simulink model "controllo_ottimo_PID"  (R2026a)
settings: Solver=VariableStepAuto  StopTime=30
values from neighbouring files (symbols this model uses):
  A = [0 0 1 0; 0 0 0 1; -2.517 0 -10.915 0; 0 0 0 0]    [sistema_lineare.m]
  B = [0 0; 0 0; 21.83 0; 0 1.236]    [sistema_lineare.m]
  C = [1 0 0 0; 0 1 0 0; 0 0 1 0; 0 0 0 1]    [sistema_lineare.m]
  D = [0 0; 0 0; 0 0; 0 0]    [sistema_lineare.m]
  u_regime = pinv(Bd) * (I - Ad) * x_f    [CONTROLLO_OTTIMO_discretizzazione_feedforward.m]
  u_star = inv(W)*Rd'*inv(Rd*inv(W)*Rd')*(x_f - Ad^n*x_0)    [CONTROLLO_OTTIMO_discretizzazione_feedforward.m]
  x_0 = [0.117; 0; 0; 0]    [CONTROLLO_OTTIMO_discretizzazione_feedforward.m]
undefined symbols (not defined in the file or in its folder): Ad, Bd
libraries: slpidlib x4
settings Model: Creator=user  LastModifiedBy=user

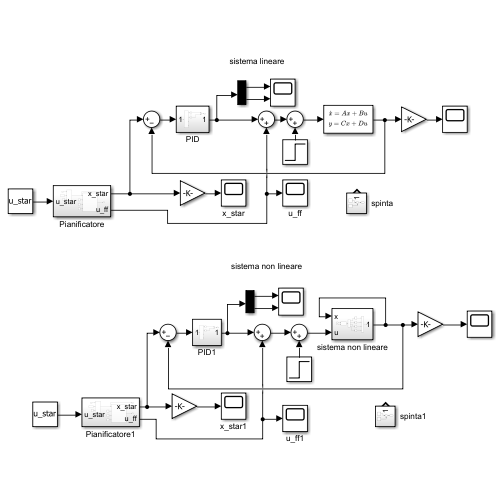
[thumbnail: Simulink's stored preview of the top-level diagram]
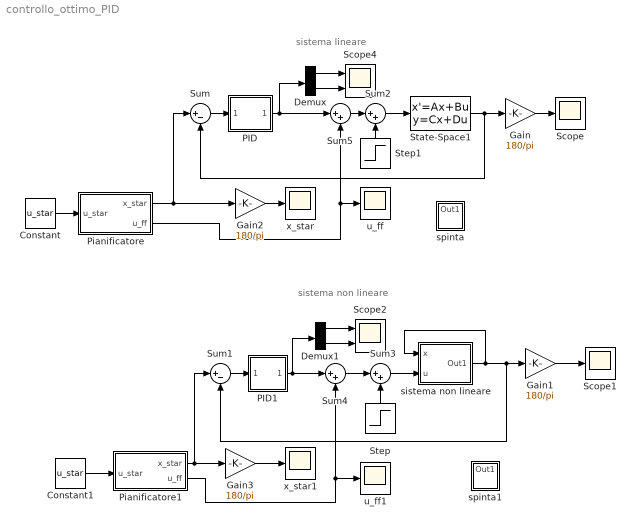
== system controllo_ottimo_PID ==
  note: sistema lineare
  note: sistema non lineare
  Constant : Constant  Value=u_star
  Constant1 : Constant  Value=u_star
  Demux : Demux  Outputs=2
  Demux1 : Demux  Outputs=2
  Gain{,1..3} (4 alike) : Gain  Gain=180/pi
  PID : Subsystem
  PID1 : Subsystem
  Pianificatore : Subsystem
  Pianificatore1 : Subsystem
  Scope : Scope
      settings: Title=angoli e velocità angolari  ActiveDisplayYMinimum=-19.863928702549515  ActiveDisplayYMaximum=100.91969713509383
  Scope1 : Scope
      settings: Title=angoli e velocità angolari  ActiveDisplayYMinimum=-19.863928702549515  ActiveDisplayYMaximum=100.91969713509383  DataLoggingVariableName=ScopeData4
  Scope2 : Scope  NumInputPorts=2
      settings: ActiveDisplayYMinimum=-3.9476866423630206  ActiveDisplayYMaximum=12.694242209293055  DataLoggingVariableName=ScopeData3
  Scope4 : Scope  NumInputPorts=2
      settings: ActiveDisplayYMinimum=-3.9476866423630206  ActiveDisplayYMaximum=12.694242209293055  DataLoggingVariableName=ScopeData6
  State-Space1 : StateSpace  A=A  B=B  C=C  D=D  InitialCondition=[0.117;0;0;0]
  Step : Step  Time=5  FinalValue=0.1  SampleTime=0
  Step1 : Step  Time=5  SampleTime=0
  Sum : Sum  Inputs=|+-
  Sum1 : Sum  Inputs=|+-
  Sum{2..5} (4 alike) : Sum  Inputs=|++
  sistema non lineare : Subsystem
  spinta : Subsystem
  spinta1 : Subsystem
  u_ff : Scope
      settings: Title=u_ff  ActiveDisplayYMinimum=-0.76735028378378445  ActiveDisplayYMaximum=0.87981383783783862
  u_ff1 : Scope
      settings: Title=u_ff  ActiveDisplayYMinimum=-0.70558162922297274  ActiveDisplayYMaximum=1.6384596207770272
  x_star : Scope
      settings: Title=x_star  ActiveDisplayYMinimum=-96.1931  ActiveDisplayYMaximum=305.783  DataLoggingVariableName=ScopeData2
  x_star1 : Scope
      settings: Title=x_star  ActiveDisplayYMinimum=-96.1931  ActiveDisplayYMaximum=305.783  DataLoggingVariableName=ScopeData2
  wires:
  Sum/1 -> PID/1(In1)
  Gain/1 -> Scope/1
  State-Space1/1 -> Sum/2, Gain/1
  Pianificatore1/2(u_ff) -> u_ff1/1, Sum4/2
  Constant1/1 -> Pianificatore1/1(u_star)
  Gain3/1 -> x_star1/1
  sistema non lineare/1(Out1) -> Gain1/1, Sum1/2, sistema non lineare/1(x)
  Sum1/1 -> PID1/1(In1)
  Pianificatore1/1(x_star) -> Gain3/1, Sum1/1
  PID1/1(Out1) -> Sum4/1, Demux1/1
  PID/1(Out1) -> Sum5/1, Demux/1
  Pianificatore/1(x_star) -> Gain2/1, Sum/1
  Gain2/1 -> x_star/1
  Sum4/1 -> Sum3/1
  Sum5/1 -> Sum2/1
  Demux/1 -> Scope4/1
  Demux/2 -> Scope4/2
  Demux1/1 -> Scope2/1
  Demux1/2 -> Scope2/2
  Step1/1 -> Sum2/2
  Step/1 -> Sum3/2
  Pianificatore/2(u_ff) -> Sum5/2, u_ff/1
  Constant/1 -> Pianificatore/1(u_star)
  Sum2/1 -> State-Space1/1
  Sum3/1 -> sistema non lineare/2(u)
  Gain1/1 -> Scope1/1

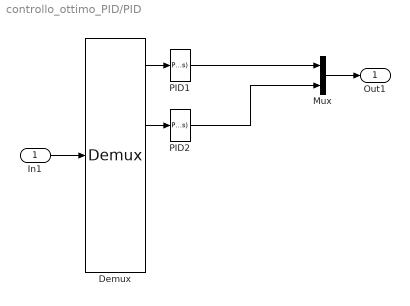
== system controllo_ottimo_PID/PID ==
  In1 : Inport
  Demux : Demux
  Mux : Mux  Inputs=2
  PID1 : slpidlib/PID Controller  Controller=PID  Form=Parallel  TimeDomain=Continuous-time  UseExternalTs=off  SampleTime=-1  IntegratorMethod=Forward Euler  FilterMethod=Forward Euler  ControllerParametersSource=internal  P=2.11205018237787  I=1.49141592854366  UseKiTs=off  D=0.250048510902589  UseExternalDerivativeSource=off  N=10  UseFilter=on  TunerSelectOption=Transfer Function Based (PID Tuner App)  InitialConditionSource=internal  InitialConditionForIntegrator=0  InitialConditionForFilter=0  DifferentiatorICPrevScaledInput=0  ExternalReset=none  TrackingMode=off  Kt=1  LimitOutput=off  SatLimitsSource=internal  UpperSaturationLimit=inf  LowerSaturationLimit=-inf  LinearizeAsGain=on  AntiWindupMode=none  Kb=1  LimitIntegrator=off  UpperIntegratorSaturationLimit=inf  LowerIntegratorSaturationLimit=-inf  POutMin=[]  POutMax=[]  IOutMin=[]  IOutMax=[]  DOutMin=[]  DOutMax=[]  NOutMin=[]  NOutMax=[]  SumOutMin=[]  SumOutMax=[]  SaturationOutMin=[]  SaturationOutMax=[]  PParamMin=[]  PParamMax=[]  IParamMin=[]  IParamMax=[]  DParamMin=[]  DParamMax=[]  NParamMin=[]  NParamMax=[]  KbParamMin=[]  KbParamMax=[]  KtParamMin=[]  KtParamMax=[]  KbOutMin=[]  KbOutMax=[]  KtOutMin=[]  KtOutMax=[]  IntegratorOutMin=[]  IntegratorOutMax=[]  FilterOutMin=[]  FilterOutMax=[]  SumI1OutMin=[]  SumI1OutMax=[]  SumI2OutMin=[]  SumI2OutMax=[]  SumI3OutMin=[]  SumI3OutMax=[]  SumI4OutMin=[]  SumI4OutMax=[]  SumDOutMin=[]  SumDOutMax=[]  DifferentiatorOutMin=[]  DifferentiatorOutMax=[]  FilterDiffOutCoefMin=[]  FilterDiffOutCoefMax=[]  ReciprocalOutMin=[]  ReciprocalOutMax=[]  SumDenOutMin=[]  SumDenOutMax=[]  SumNumOutMin=[]  SumNumOutMax=[]  DivideOutMin=[]  DivideOutMax=[]  UdiffTsProdOutMin=[]  UdiffTsProdOutMax=[]  NTsProdOutMin=[]  NTsProdOutMax=[]  UintegralTsProdOutMin=[]  UintegralTsProdOutMax=[]  UngainTsProdOutMin=[]  UngainTsProdOutMax=[]  ClampingZeroOutDataTypeStr=Inherit: Inherit via back propagation  ClampingZeroOutMin=[]  ClampingZeroOutMax=[]  FilterDenConstantOutDataTypeStr=Inherit: Inherit via back propagation  FilterDenConstantOutMin=[]  FilterDenConstantOutMax=[]  PCopyOutDataTypeStr=Inherit: Inherit via back propagation  PCopyOutMin=[]  PCopyOutMax=[]  NCopyOutDataTypeStr=Inherit: Inherit via back propagation  NCopyOutMin=[]  NCopyOutMax=[]  IntegratorContinuousStateAttributes=''  IntegratorStateMustResolveToSignalObject=off  IntegratorRTWStateStorageClass=Auto  FilterContinuousStateAttributes=''  FilterStateMustResolveToSignalObject=off  FilterRTWStateStorageClass=Auto  ParallelPVariant=InternalParameters  IdealPVariant=Disabled  IVariant=InternalParameters  DVariant=InternalParameters  IntegratorVariant=Continuous  SatVariant=Disabled  AWVariant=Passthrough  PCopyVariant=Disabled  TRVariant=Disabled  FdbkBlocksVariant=Forward  IdealPFdbkVariant=Disabled  SatFdbkVariant=Disabled  DerivativeFilterVariant=ContFilter  NVariant=InternalParameters  NCopyVariant=Disabled  FilterICVariant=InternalICsFilter  IntegratorICVariant=InternalICs  ExternalResetVariant=Disabled  TRSumVariant=Passthrough  SumFdbkVariant=Disabled  SumVariant=Sum_PID  TsampFilterVariant=InternalTs  TsampNgainVariant=Passthrough  TsampIntegralVariant=Disabled_SignalSpec  ExternalSaturationOutDataTypeStr=Inherit: Same as second input  DerivativeSourceVariant=ErrorSignal  PreIntVariant=InternalPreInt
  PID2 : slpidlib/PID Controller  Controller=PID  Form=Parallel  TimeDomain=Continuous-time  UseExternalTs=off  SampleTime=-1  IntegratorMethod=Forward Euler  FilterMethod=Forward Euler  ControllerParametersSource=internal  P=15.4746759421667  I=7.38828621314958  UseKiTs=off  D=7.89104179263979  UseExternalDerivativeSource=off  N=10  UseFilter=on  TunerSelectOption=Transfer Function Based (PID Tuner App)  InitialConditionSource=internal  InitialConditionForIntegrator=0  InitialConditionForFilter=0  DifferentiatorICPrevScaledInput=0  ExternalReset=none  TrackingMode=off  Kt=1  LimitOutput=off  SatLimitsSource=internal  UpperSaturationLimit=inf  LowerSaturationLimit=-inf  LinearizeAsGain=on  AntiWindupMode=none  Kb=1  LimitIntegrator=off  UpperIntegratorSaturationLimit=inf  LowerIntegratorSaturationLimit=-inf  POutMin=[]  POutMax=[]  IOutMin=[]  IOutMax=[]  DOutMin=[]  DOutMax=[]  NOutMin=[]  NOutMax=[]  SumOutMin=[]  SumOutMax=[]  SaturationOutMin=[]  SaturationOutMax=[]  PParamMin=[]  PParamMax=[]  IParamMin=[]  IParamMax=[]  DParamMin=[]  DParamMax=[]  NParamMin=[]  NParamMax=[]  KbParamMin=[]  KbParamMax=[]  KtParamMin=[]  KtParamMax=[]  KbOutMin=[]  KbOutMax=[]  KtOutMin=[]  KtOutMax=[]  IntegratorOutMin=[]  IntegratorOutMax=[]  FilterOutMin=[]  FilterOutMax=[]  SumI1OutMin=[]  SumI1OutMax=[]  SumI2OutMin=[]  SumI2OutMax=[]  SumI3OutMin=[]  SumI3OutMax=[]  SumI4OutMin=[]  SumI4OutMax=[]  SumDOutMin=[]  SumDOutMax=[]  DifferentiatorOutMin=[]  DifferentiatorOutMax=[]  FilterDiffOutCoefMin=[]  FilterDiffOutCoefMax=[]  ReciprocalOutMin=[]  ReciprocalOutMax=[]  SumDenOutMin=[]  SumDenOutMax=[]  SumNumOutMin=[]  SumNumOutMax=[]  DivideOutMin=[]  DivideOutMax=[]  UdiffTsProdOutMin=[]  UdiffTsProdOutMax=[]  NTsProdOutMin=[]  NTsProdOutMax=[]  UintegralTsProdOutMin=[]  UintegralTsProdOutMax=[]  UngainTsProdOutMin=[]  UngainTsProdOutMax=[]  ClampingZeroOutDataTypeStr=Inherit: Inherit via back propagation  ClampingZeroOutMin=[]  ClampingZeroOutMax=[]  FilterDenConstantOutDataTypeStr=Inherit: Inherit via back propagation  FilterDenConstantOutMin=[]  FilterDenConstantOutMax=[]  PCopyOutDataTypeStr=Inherit: Inherit via back propagation  PCopyOutMin=[]  PCopyOutMax=[]  NCopyOutDataTypeStr=Inherit: Inherit via back propagation  NCopyOutMin=[]  NCopyOutMax=[]  IntegratorContinuousStateAttributes=''  IntegratorStateMustResolveToSignalObject=off  IntegratorRTWStateStorageClass=Auto  FilterContinuousStateAttributes=''  FilterStateMustResolveToSignalObject=off  FilterRTWStateStorageClass=Auto  ParallelPVariant=InternalParameters  IdealPVariant=Disabled  IVariant=InternalParameters  DVariant=InternalParameters  IntegratorVariant=Continuous  SatVariant=Disabled  AWVariant=Passthrough  PCopyVariant=Disabled  TRVariant=Disabled  FdbkBlocksVariant=Forward  IdealPFdbkVariant=Disabled  SatFdbkVariant=Disabled  DerivativeFilterVariant=ContFilter  NVariant=InternalParameters  NCopyVariant=Disabled  FilterICVariant=InternalICsFilter  IntegratorICVariant=InternalICs  ExternalResetVariant=Disabled  TRSumVariant=Passthrough  SumFdbkVariant=Disabled  SumVariant=Sum_PID  TsampFilterVariant=InternalTs  TsampNgainVariant=Passthrough  TsampIntegralVariant=Disabled_SignalSpec  ExternalSaturationOutDataTypeStr=Inherit: Same as second input  DerivativeSourceVariant=ErrorSignal  PreIntVariant=InternalPreInt
  Out1 : Outport
  wires:
  In1/1 -> Demux/1
  Demux/1 -> PID1/1
  Demux/2 -> PID2/1
  Mux/1 -> Out1/1
  PID2/1 -> Mux/2
  PID1/1 -> Mux/1

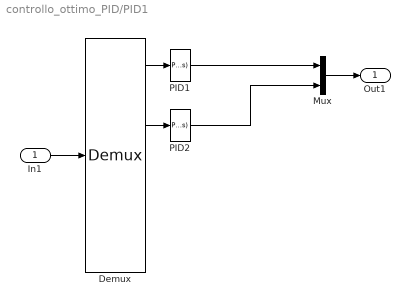
== system controllo_ottimo_PID/PID1 ==
  In1 : Inport
  Demux : Demux
  Mux : Mux  Inputs=2
  PID1 : slpidlib/PID Controller  Controller=PID  Form=Parallel  TimeDomain=Continuous-time  UseExternalTs=off  SampleTime=-1  IntegratorMethod=Forward Euler  FilterMethod=Forward Euler  ControllerParametersSource=internal  P=2.11205018237787  I=1.49141592854366  UseKiTs=off  D=0.250048510902589  UseExternalDerivativeSource=off  N=10  UseFilter=on  TunerSelectOption=Transfer Function Based (PID Tuner App)  InitialConditionSource=internal  InitialConditionForIntegrator=0  InitialConditionForFilter=0  DifferentiatorICPrevScaledInput=0  ExternalReset=none  TrackingMode=off  Kt=1  LimitOutput=off  SatLimitsSource=internal  UpperSaturationLimit=inf  LowerSaturationLimit=-inf  LinearizeAsGain=on  AntiWindupMode=none  Kb=1  LimitIntegrator=off  UpperIntegratorSaturationLimit=inf  LowerIntegratorSaturationLimit=-inf  POutMin=[]  POutMax=[]  IOutMin=[]  IOutMax=[]  DOutMin=[]  DOutMax=[]  NOutMin=[]  NOutMax=[]  SumOutMin=[]  SumOutMax=[]  SaturationOutMin=[]  SaturationOutMax=[]  PParamMin=[]  PParamMax=[]  IParamMin=[]  IParamMax=[]  DParamMin=[]  DParamMax=[]  NParamMin=[]  NParamMax=[]  KbParamMin=[]  KbParamMax=[]  KtParamMin=[]  KtParamMax=[]  KbOutMin=[]  KbOutMax=[]  KtOutMin=[]  KtOutMax=[]  IntegratorOutMin=[]  IntegratorOutMax=[]  FilterOutMin=[]  FilterOutMax=[]  SumI1OutMin=[]  SumI1OutMax=[]  SumI2OutMin=[]  SumI2OutMax=[]  SumI3OutMin=[]  SumI3OutMax=[]  SumI4OutMin=[]  SumI4OutMax=[]  SumDOutMin=[]  SumDOutMax=[]  DifferentiatorOutMin=[]  DifferentiatorOutMax=[]  FilterDiffOutCoefMin=[]  FilterDiffOutCoefMax=[]  ReciprocalOutMin=[]  ReciprocalOutMax=[]  SumDenOutMin=[]  SumDenOutMax=[]  SumNumOutMin=[]  SumNumOutMax=[]  DivideOutMin=[]  DivideOutMax=[]  UdiffTsProdOutMin=[]  UdiffTsProdOutMax=[]  NTsProdOutMin=[]  NTsProdOutMax=[]  UintegralTsProdOutMin=[]  UintegralTsProdOutMax=[]  UngainTsProdOutMin=[]  UngainTsProdOutMax=[]  ClampingZeroOutDataTypeStr=Inherit: Inherit via back propagation  ClampingZeroOutMin=[]  ClampingZeroOutMax=[]  FilterDenConstantOutDataTypeStr=Inherit: Inherit via back propagation  FilterDenConstantOutMin=[]  FilterDenConstantOutMax=[]  PCopyOutDataTypeStr=Inherit: Inherit via back propagation  PCopyOutMin=[]  PCopyOutMax=[]  NCopyOutDataTypeStr=Inherit: Inherit via back propagation  NCopyOutMin=[]  NCopyOutMax=[]  IntegratorContinuousStateAttributes=''  IntegratorStateMustResolveToSignalObject=off  IntegratorRTWStateStorageClass=Auto  FilterContinuousStateAttributes=''  FilterStateMustResolveToSignalObject=off  FilterRTWStateStorageClass=Auto  ParallelPVariant=InternalParameters  IdealPVariant=Disabled  IVariant=InternalParameters  DVariant=InternalParameters  IntegratorVariant=Continuous  SatVariant=Disabled  AWVariant=Passthrough  PCopyVariant=Disabled  TRVariant=Disabled  FdbkBlocksVariant=Forward  IdealPFdbkVariant=Disabled  SatFdbkVariant=Disabled  DerivativeFilterVariant=ContFilter  NVariant=InternalParameters  NCopyVariant=Disabled  FilterICVariant=InternalICsFilter  IntegratorICVariant=InternalICs  ExternalResetVariant=Disabled  TRSumVariant=Passthrough  SumFdbkVariant=Disabled  SumVariant=Sum_PID  TsampFilterVariant=InternalTs  TsampNgainVariant=Passthrough  TsampIntegralVariant=Disabled_SignalSpec  ExternalSaturationOutDataTypeStr=Inherit: Same as second input  DerivativeSourceVariant=ErrorSignal  PreIntVariant=InternalPreInt
  PID2 : slpidlib/PID Controller  Controller=PID  Form=Parallel  TimeDomain=Continuous-time  UseExternalTs=off  SampleTime=-1  IntegratorMethod=Forward Euler  FilterMethod=Forward Euler  ControllerParametersSource=internal  P=15.4746759421667  I=7.38828621314958  UseKiTs=off  D=7.89104179263979  UseExternalDerivativeSource=off  N=10  UseFilter=on  TunerSelectOption=Transfer Function Based (PID Tuner App)  InitialConditionSource=internal  InitialConditionForIntegrator=0  InitialConditionForFilter=0  DifferentiatorICPrevScaledInput=0  ExternalReset=none  TrackingMode=off  Kt=1  LimitOutput=off  SatLimitsSource=internal  UpperSaturationLimit=inf  LowerSaturationLimit=-inf  LinearizeAsGain=on  AntiWindupMode=none  Kb=1  LimitIntegrator=off  UpperIntegratorSaturationLimit=inf  LowerIntegratorSaturationLimit=-inf  POutMin=[]  POutMax=[]  IOutMin=[]  IOutMax=[]  DOutMin=[]  DOutMax=[]  NOutMin=[]  NOutMax=[]  SumOutMin=[]  SumOutMax=[]  SaturationOutMin=[]  SaturationOutMax=[]  PParamMin=[]  PParamMax=[]  IParamMin=[]  IParamMax=[]  DParamMin=[]  DParamMax=[]  NParamMin=[]  NParamMax=[]  KbParamMin=[]  KbParamMax=[]  KtParamMin=[]  KtParamMax=[]  KbOutMin=[]  KbOutMax=[]  KtOutMin=[]  KtOutMax=[]  IntegratorOutMin=[]  IntegratorOutMax=[]  FilterOutMin=[]  FilterOutMax=[]  SumI1OutMin=[]  SumI1OutMax=[]  SumI2OutMin=[]  SumI2OutMax=[]  SumI3OutMin=[]  SumI3OutMax=[]  SumI4OutMin=[]  SumI4OutMax=[]  SumDOutMin=[]  SumDOutMax=[]  DifferentiatorOutMin=[]  DifferentiatorOutMax=[]  FilterDiffOutCoefMin=[]  FilterDiffOutCoefMax=[]  ReciprocalOutMin=[]  ReciprocalOutMax=[]  SumDenOutMin=[]  SumDenOutMax=[]  SumNumOutMin=[]  SumNumOutMax=[]  DivideOutMin=[]  DivideOutMax=[]  UdiffTsProdOutMin=[]  UdiffTsProdOutMax=[]  NTsProdOutMin=[]  NTsProdOutMax=[]  UintegralTsProdOutMin=[]  UintegralTsProdOutMax=[]  UngainTsProdOutMin=[]  UngainTsProdOutMax=[]  ClampingZeroOutDataTypeStr=Inherit: Inherit via back propagation  ClampingZeroOutMin=[]  ClampingZeroOutMax=[]  FilterDenConstantOutDataTypeStr=Inherit: Inherit via back propagation  FilterDenConstantOutMin=[]  FilterDenConstantOutMax=[]  PCopyOutDataTypeStr=Inherit: Inherit via back propagation  PCopyOutMin=[]  PCopyOutMax=[]  NCopyOutDataTypeStr=Inherit: Inherit via back propagation  NCopyOutMin=[]  NCopyOutMax=[]  IntegratorContinuousStateAttributes=''  IntegratorStateMustResolveToSignalObject=off  IntegratorRTWStateStorageClass=Auto  FilterContinuousStateAttributes=''  FilterStateMustResolveToSignalObject=off  FilterRTWStateStorageClass=Auto  ParallelPVariant=InternalParameters  IdealPVariant=Disabled  IVariant=InternalParameters  DVariant=InternalParameters  IntegratorVariant=Continuous  SatVariant=Disabled  AWVariant=Passthrough  PCopyVariant=Disabled  TRVariant=Disabled  FdbkBlocksVariant=Forward  IdealPFdbkVariant=Disabled  SatFdbkVariant=Disabled  DerivativeFilterVariant=ContFilter  NVariant=InternalParameters  NCopyVariant=Disabled  FilterICVariant=InternalICsFilter  IntegratorICVariant=InternalICs  ExternalResetVariant=Disabled  TRSumVariant=Passthrough  SumFdbkVariant=Disabled  SumVariant=Sum_PID  TsampFilterVariant=InternalTs  TsampNgainVariant=Passthrough  TsampIntegralVariant=Disabled_SignalSpec  ExternalSaturationOutDataTypeStr=Inherit: Same as second input  DerivativeSourceVariant=ErrorSignal  PreIntVariant=InternalPreInt
  Out1 : Outport
  wires:
  In1/1 -> Demux/1
  Demux/1 -> PID1/1
  Demux/2 -> PID2/1
  Mux/1 -> Out1/1
  PID2/1 -> Mux/2
  PID1/1 -> Mux/1

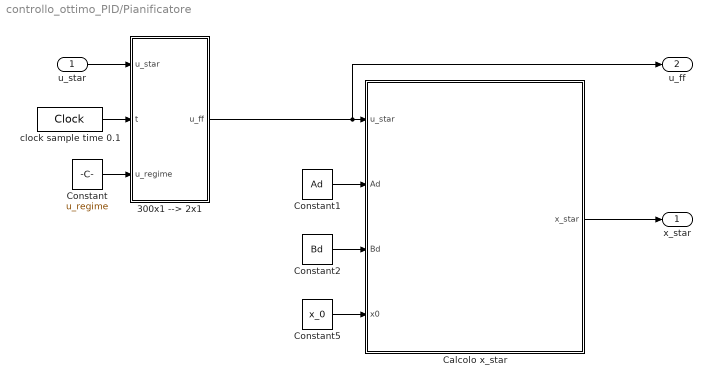
== system controllo_ottimo_PID/Pianificatore ==
  u_star : Inport
  300x1 --> 2x1 : MATLAB Function  TreatAsAtomicUnit=on
  Calcolo x_star : MATLAB Function  TreatAsAtomicUnit=on
  Constant : Constant  Value=u_regime
  Constant1 : Constant  Value=Ad
  Constant2 : Constant  Value=Bd
  Constant5 : Constant  Value=x_0
  clock sample time 0.1 : DigitalClock  SampleTime=0.1
  x_star : Outport
  u_ff : Outport  Port=2
  wires:
  clock sample time 0.1/1 -> 300x1 --> 2x1/2(t)
  300x1 --> 2x1/1(u_ff) -> u_ff/1, Calcolo x_star/1(u_star)
  Constant5/1 -> Calcolo x_star/4(x0)
  Constant2/1 -> Calcolo x_star/3(Bd)
  Constant1/1 -> Calcolo x_star/2(Ad)
  u_star/1 -> 300x1 --> 2x1/1(u_star)
  Calcolo x_star/1(x_star) -> x_star/1
  Constant/1 -> 300x1 --> 2x1/3(u_regime)

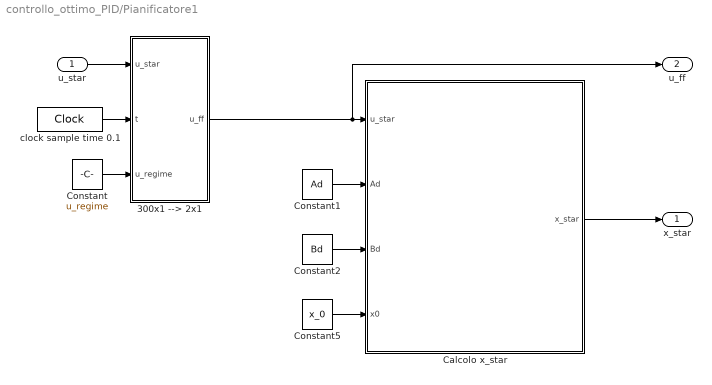
== system controllo_ottimo_PID/Pianificatore1 ==
  u_star : Inport
  300x1 --> 2x1 : MATLAB Function  TreatAsAtomicUnit=on
  Calcolo x_star : MATLAB Function  TreatAsAtomicUnit=on
  Constant : Constant  Value=u_regime
  Constant1 : Constant  Value=Ad
  Constant2 : Constant  Value=Bd
  Constant5 : Constant  Value=x_0
  clock sample time 0.1 : DigitalClock  SampleTime=0.1
  x_star : Outport
  u_ff : Outport  Port=2
  wires:
  clock sample time 0.1/1 -> 300x1 --> 2x1/2(t)
  300x1 --> 2x1/1(u_ff) -> u_ff/1, Calcolo x_star/1(u_star)
  Constant5/1 -> Calcolo x_star/4(x0)
  Constant2/1 -> Calcolo x_star/3(Bd)
  Constant1/1 -> Calcolo x_star/2(Ad)
  u_star/1 -> 300x1 --> 2x1/1(u_star)
  Calcolo x_star/1(x_star) -> x_star/1
  Constant/1 -> 300x1 --> 2x1/3(u_regime)

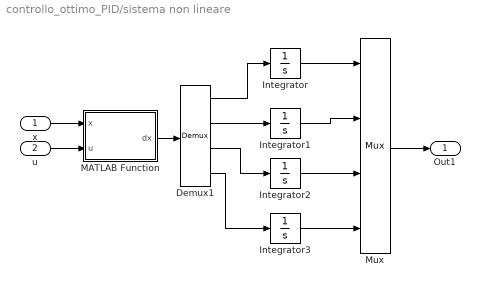
== system controllo_ottimo_PID/sistema non lineare ==
  x : Inport
  u : Inport  Port=2
  Demux1 : Demux
  Integrator : Integrator  InitialCondition=0.117
  Integrator1 : Integrator
  Integrator2 : Integrator
  Integrator3 : Integrator
  MATLAB Function : MATLAB Function  TreatAsAtomicUnit=on
  Mux : Mux
  Out1 : Outport  PortDimensions=4
  wires:
  MATLAB Function/1(dx) -> Demux1/1
  Demux1/1 -> Integrator/1
  Demux1/2 -> Integrator1/1
  Mux/1 -> Out1/1
  x/1 -> MATLAB Function/1(x)
  u/1 -> MATLAB Function/2(u)
  Integrator/1 -> Mux/1
  Integrator1/1 -> Mux/2
  Integrator3/1 -> Mux/4
  Integrator2/1 -> Mux/3
  Demux1/3 -> Integrator2/1
  Demux1/4 -> Integrator3/1

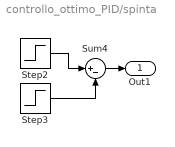
== system controllo_ottimo_PID/spinta ==
  Step2 : Step  Time=20  SampleTime=0
  Step3 : Step  Time=20.1  SampleTime=0
  Sum4 : Sum  Inputs=|+-
  Out1 : Outport
  wires:
  Step3/1 -> Sum4/2
  Step2/1 -> Sum4/1
  Sum4/1 -> Out1/1

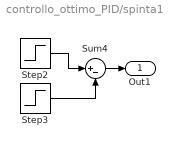
== system controllo_ottimo_PID/spinta1 ==
  Step2 : Step  Time=20  SampleTime=0
  Step3 : Step  Time=20.1  SampleTime=0
  Sum4 : Sum  Inputs=|+-
  Out1 : Outport
  wires:
  Step3/1 -> Sum4/2
  Step2/1 -> Sum4/1
  Sum4/1 -> Out1/1

== matlab function controllo_ottimo_PID/Pianificatore/300x1 --> 2x1 ==
  data: u_star input; t input; u_ff output; u_regime input
function u_ff = fcn(u_star, t, u_regime)
    m = 2;  % Num righe in uscita
    Ts=0.1;  % Tempo di campionamento

    % Inizializziamo u_ff come un vettore colonna FISSO 2x1
    u_ff = zeros(m, 1); 
    
    n_steps = length(u_star) / m;
    k = floor(t / Ts);
    
    if k >= 0 && k < n_steps
        idx_inizio = k * m + 1;
        % Estraiamo i dati
        u_temp = u_star(idx_inizio : idx_inizio + m - 1);
        % Assegniamo i valori al vettore pre-allocato
        u_ff(1) = u_temp(1);
        u_ff(2) = u_temp(2);
    else
        % --- FASE 2: IL REGIME (Da k=150 in poi all'infinito) ---
        % Qui comanda u_regime
        u_ff(1) = u_regime(1);
        u_ff(2) = u_regime(2);
    end
end

== matlab function controllo_ottimo_PID/sistema non lineare/MATLAB Function ==
  data: x input; u input; dx output
function dx = trms_dynamics(x, u)
    % Estrazione degli stati dal vettore x
    x1 = x(1);
    x2 = x(2);
    x3 = x(3);
    x4 = x(4);
    
    % Estrazione degli ingressi dal vettore u
    u1 = u(1);
    u2 = u(2);
    
    % Calcolo delle equazioni differenziali
    dx1 = x3;
    dx2 = x4;
    
    % Dinamica di x3
    dx3 = 21.83 * (0.0981*cos(x1) - 0.833*sin(x1) + u1 - 0.195*(x4^2)*sin(x1)*cos(x1) - 0.5*x3);
    
    % Dinamica di x4 (divisa in numeratore e denominatore per chiarezza)
    num_dx4 = u2*cos(x1) - 0.01*x4;
    den_dx4 = 0.01667*(sin(x1)^2) + 0.03728*(cos(x1)^2) + 0.00015;
    dx4 = num_dx4 / den_dx4;
    
    % Vettore colonna delle derivate
    dx = [dx1; dx2; dx3; dx4];
end

== matlab function controllo_ottimo_PID/Pianificatore/Calcolo x_star ==
  settings: updateMethod=DISCRETE  sampleTime=0.1
  data: u_star input; x_star output; Ad input; Bd input; x0 input
function x_star = fcn(u_star, Ad, Bd, x0)
    % u_star: ingresso ottimo attuale (2x1)
    % Ad: 4x4, Bd: 4x2
    
    persistent x_state;
    
    % Inizializzazione al primo passo
    if isempty(x_state)
        x_state = x0;
    end
    
    % L'uscita della funzione è lo stato attuale
    x_star = x_state;
    
    % Aggiornamento per il prossimo passo k+1
    % x_star(k+1) = Ad*x_star(k) + Bd*u_star(k)
    x_state = Ad * x_state + Bd * u_star;
end

== matlab function controllo_ottimo_PID/Pianificatore1/300x1 --> 2x1 ==
  data: u_star input; t input; u_ff output; u_regime input
function u_ff = fcn(u_star, t, u_regime)
    m = 2;  % Num righe in uscita
    Ts=0.1;  % Tempo di campionamento

    % Inizializziamo u_ff come un vettore colonna FISSO 2x1
    u_ff = zeros(m, 1); 
    
    n_steps = length(u_star) / m;
    k = floor(t / Ts);
    
    if k >= 0 && k < n_steps
        idx_inizio = k * m + 1;
        % Estraiamo i dati
        u_temp = u_star(idx_inizio : idx_inizio + m - 1);
        % Assegniamo i valori al vettore pre-allocato
        u_ff(1) = u_temp(1);
        u_ff(2) = u_temp(2);
    else
        % --- FASE 2: IL REGIME (Da k=150 in poi all'infinito) ---
        % Qui comanda u_regime
        u_ff(1) = u_regime(1);
        u_ff(2) = u_regime(2);
    end
end

== matlab function controllo_ottimo_PID/Pianificatore1/Calcolo x_star ==
  settings: updateMethod=DISCRETE  sampleTime=0.1
  data: u_star input; x_star output; Ad input; Bd input; x0 input
function x_star = fcn(u_star, Ad, Bd, x0)
    % u_star: ingresso ottimo attuale (2x1)
    % Ad: 4x4, Bd: 4x2
    
    persistent x_state;
    
    % Inizializzazione al primo passo
    if isempty(x_state)
        x_state = x0;
    end
    
    % L'uscita della funzione è lo stato attuale
    x_star = x_state;
    
    % Aggiornamento per il prossimo passo k+1
    % x_star(k+1) = Ad*x_star(k) + Bd*u_star(k)
    x_state = Ad * x_state + Bd * u_star;
end
